simulink model "R3_2"  (R2016a)
settings: Solver=VariableStepAuto  StartTime=0.0  StopTime=8  RelTol=1e-3
settings Model: Creator=NAD  LastModifiedBy=NAD

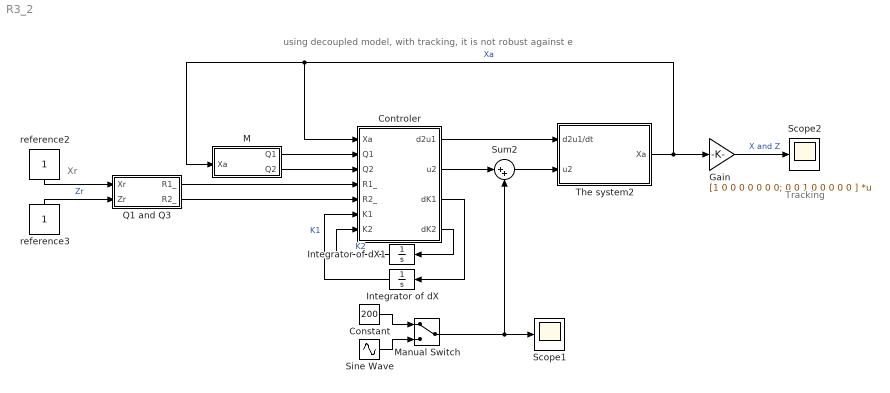
== system R3_2 ==
  note: Xr
  note: Tracking
  note: using decoupled model, with tracking, it is not robust against e
  Constant : Constant  Value=200
  Controler : MATLAB Function  TreatAsAtomicUnit=on
  Gain : Gain  Gain=[1 0 0 0 0 0 0 0; 0 0 1 0 0 0 0 0 ]  Multiplication=Matrix(K*u) (u vector)
  Integrator of dX : Integrator  InitialCondition=10
  Integrator of dX1 : Integrator  InitialCondition=10
  M : MATLAB Function  TreatAsAtomicUnit=on
  Manual Switch : ManualSwitch
  Q1 and Q3 : Subsystem
  Scope1 : Scope
  Scope2 : Scope
  Sine Wave : Sin  Amplitude=200  SampleTime=0
  Sum2 : Sum  Inputs=|++
  The system2 : Subsystem
  reference2 : Constant
  reference3 : Constant
  wires:
  The system2/1(Xa) -> Gain/1, M/1(Xa), Controler/1(Xa)  "Xa"
  M/1(Q1) -> Controler/2(Q1)
  M/2(Q2) -> Controler/3(Q2)
  Controler/1(d2u1) -> The system2/1(d2u1/dt)
  Controler/2(u2) -> Sum2/1
  Sum2/1 -> The system2/2(u2)
  Manual Switch/1 -> Sum2/2, Scope1/1
  Q1 and Q3/2(R2_) -> Controler/5(R2_)
  Q1 and Q3/1(R1_) -> Controler/4(R1_)
  Gain/1 -> Scope2/1  "X and Z"
  Controler/3(dK1) -> Integrator of dX/1
  Integrator of dX/1 -> Controler/6(K1)  "K1"
  Controler/4(dK2) -> Integrator of dX1/1
  Integrator of dX1/1 -> Controler/7(K2)  "K2"
  Constant/1 -> Manual Switch/1
  Sine Wave/1 -> Manual Switch/2
  reference2/1 -> Q1 and Q3/1(Xr)
  reference3/1 -> Q1 and Q3/2(Zr)  "Zr"

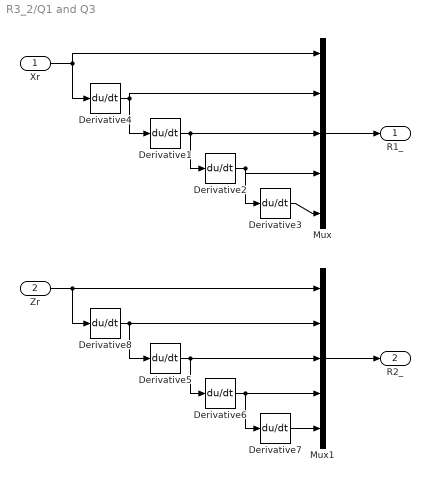
== system R3_2/Q1 and Q3 ==
  Xr : Inport
  Zr : Inport  Port=2
  Derivative{1..8} (8 alike) : Derivative
  Mux : Mux  Inputs=5
  Mux1 : Mux  Inputs=5
  R1_ : Outport
  R2_ : Outport  Port=2
  wires:
  Xr/1 -> Mux/1, Derivative4/1
  Derivative1/1 -> Mux/3, Derivative2/1
  Derivative2/1 -> Derivative3/1, Mux/4
  Derivative3/1 -> Mux/5
  Derivative4/1 -> Derivative1/1, Mux/2
  Mux/1 -> R1_/1
  Zr/1 -> Derivative8/1, Mux1/1
  Derivative5/1 -> Derivative6/1, Mux1/3
  Derivative6/1 -> Derivative7/1, Mux1/4
  Derivative7/1 -> Mux1/5
  Derivative8/1 -> Mux1/2, Derivative5/1
  Mux1/1 -> R2_/1

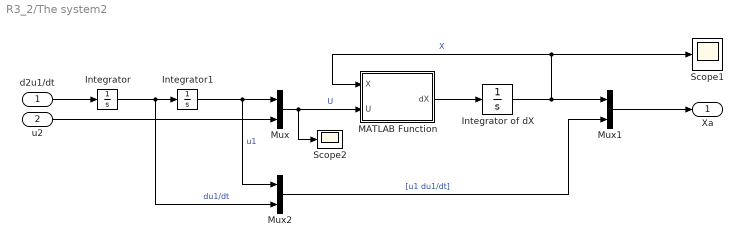
== system R3_2/The system2 ==
  d2u1/dt : Inport
  u2 : Inport  Port=2
  Integrator : Integrator
  Integrator of dX : Integrator  InitialCondition=[1 1 1 1 1 1]*0
  Integrator1 : Integrator  InitialCondition=0.1
  MATLAB Function : MATLAB Function  TreatAsAtomicUnit=on
  Mux : Mux  Inputs=2
  Mux1 : Mux  Inputs=2
  Mux2 : Mux  Inputs=2
  Scope1 : Scope
  Scope2 : Scope
  Xa : Outport
  wires:
  MATLAB Function/1(dX) -> Integrator of dX/1
  Integrator of dX/1 -> MATLAB Function/1(X), Scope1/1, Mux1/1  "X"
  Integrator/1 -> Mux2/2, Integrator1/1  "du1/dt"
  d2u1/dt/1 -> Integrator/1
  Integrator1/1 -> Mux2/1, Mux/1  "u1"
  u2/1 -> Mux/2
  Mux/1 -> Scope2/1, MATLAB Function/2(U)  "U"
  Mux1/1 -> Xa/1
  Mux2/1 -> Mux1/2  "[u1 du1/dt]"

== matlab function R3_2/M ==
  data: Xa input size=8; Q1 output size=4; Q2 output size=4
function [Q1,Q2]= fcn(Xa)
%% Definion of parameters:
x1 = Xa(1);
x2 = Xa(2);
x3 = Xa(3);
x4 = Xa(4);
x5 = Xa(5);
x6 = Xa(6);
x7 = Xa(7);
x8 = Xa(8);

%% Q1
q11 = x1;
q12=x2; 
q13 = -x7*sin(x5);
q14 = -x8*sin(x5)-x7*cos(x5)*x6;
Q1 = [q11 q12 q13 q14]';

%% Q2
q21 = x3;
q22=x4; 
q23 = cos(x5)*x7-1;
q24 = x8*cos(x5)-x7*sin(x5)*x6;
Q2 = [q21 q22 q23 q24]';

== matlab function R3_2/Controler ==
  data: Xa input size=8; Q1 input size=4; Q2 input size=4; d2u1 output size=1; R1_ input size=5; u2 output size=1; R2_ input size=5; K1 input size=1; dK1 output size=1; K2 input; dK2 output
function [d2u1,u2,dK1,dK2]= fcn(Xa,Q1,Q2,R1_,R2_,K1,K2)
%% Definion of parameters:
x1 = Xa(1);
x2 = Xa(2);
x3 = Xa(3);
x4 = Xa(4);
x5 = Xa(5);
x6 = Xa(6);
x7 = Xa(7);
x8 = Xa(8);
R1 = R1_(1:4); d4r1 = R1_(5);
R2 = R2_(1:4); d4r2 = R2_(5);

%% The surfaces:
p = 3 ;
% (s+p)^3= s^3 + 3*p*s^2 + 3*p^2.s +p^3
L = [p^3 3*p^2 3*p 1]; L_ = [0 p^3 3*p^2 3*p];
s1 = L*(Q1-R1);
s2 = L*(Q2-R2);

%% The gain (K1) dynamic:

 K1_ =300 ;
 mu1 = 10;
 eta1 = 10;
 dK1 = 0 ;
 if(K1>eta1)
     dK1 = K1_*abs(s1)*sign(abs(s1)-mu1);
 else 
     dK1 = eta1;
 end
 %% The gain (K2) dynamic:

 K2_ =300 ;
 mu2 = 10 ;
 eta2 = 10 ;
 dK2 = 0 ;
 if(K2>eta2)
     dK2 = K2_*abs(s2)*sign(abs(s2)-mu2);
 else 
     dK2 = eta2;
 end
 %% The Sliding Mode:
 W1 = -K1*sign(s1) + d4r1 - L_*(Q1-R1);
 W2 = -K2*sign(s2) + d4r2 - L_*(Q2-R2);
 W = [W1;W2] ;
 
%% The cintrol U_= [d2U1/dt; U2]: 
alpha_ = [-2*x8*cos(x5)*x6+x7*sin(x5)*x6^2
          -2*x8*sin(x5)*x6-x7*cos(x5)*x6^2];
beta_ = [-sin(x5) , -x7*cos(x5)
       cos(x5) , -x7*sin(x5)];

U_= beta_\(W-alpha_);
d2u1 = U_(1);
u2 = U_(2);

== matlab function R3_2/The system2/MATLAB Function ==
  data: X input size=6; dX output size=6; U input size=2
function dX = fcn(X,U)
%% Definion of parameters:
x1 = X(1);
x2 = X(2);
x3 = X(3);
x4 = X(4);
x5 = X(5);
x6 = X(6);

u1 = U(1);
u2 = U(2);

e = 1e-3;
%% The system:
dX = [x2
    -sin(x5)*u1 + e*cos(x5)*u2
    x4
    cos(x5)*u1 + e*sin(x5)*u2-1
    x6
    u2 ];
